simulink model "screening_stage1_pipeline"  (R2026a)
settings: Solver=VariableStepAuto
values from neighbouring files (symbols this model uses):
  m = result.lesionMasks.(code)    [runScreeningPipeline.m]
undefined symbols (not defined in the file or in its folder): n
settings Model: Creator=keert  LastModifiedBy=keert

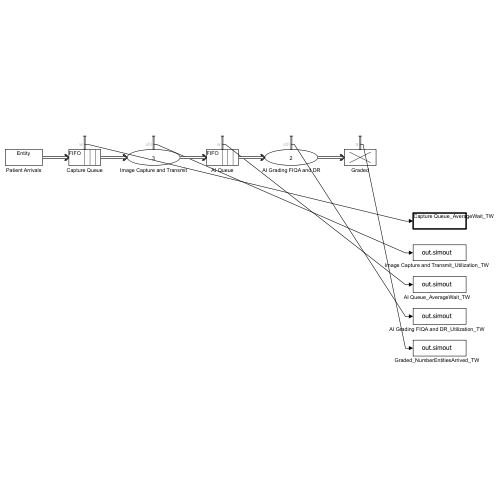
[thumbnail: Simulink's stored preview of the top-level diagram]
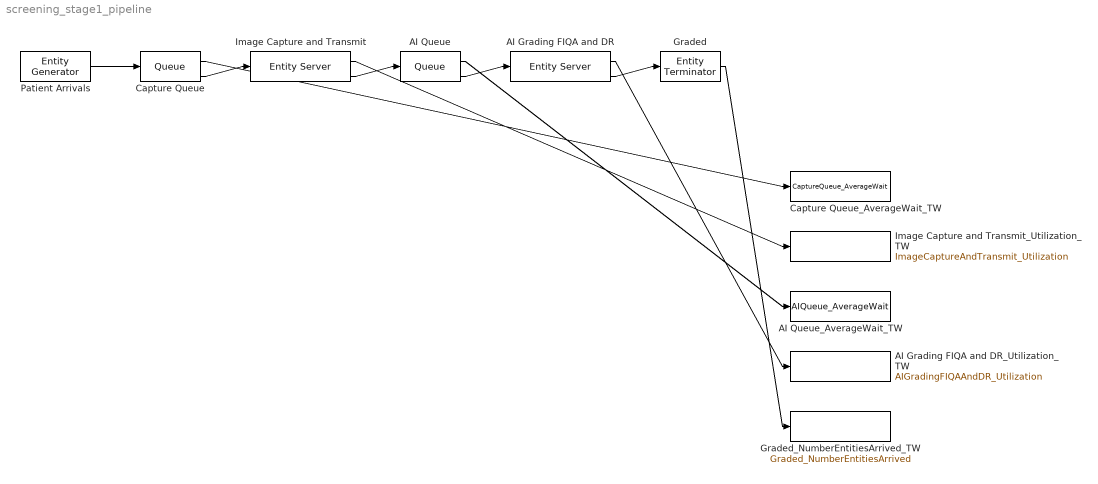
== system screening_stage1_pipeline ==
  AI Grading FIQA and DR : EntityServer  InputPortMessageModes=m  OutputPortMessageModes=n,m  Capacity=2  ServiceTimeValue=0.2  Utilization=on
      settings: OutputPortMap=o5,o9
  AI Grading FIQA and DR_Utilization_TW : ToWorkspace  VariableName=AIGradingFIQAAndDR_Utilization  SaveFormat=Structure  SampleTime=-1
  AI Queue : Queue  InputPortMessageModes=m  OutputPortMessageModes=n,m  AverageWait=on
      settings: OutputPortMap=o2,o5
  AI Queue_AverageWait_TW : ToWorkspace  VariableName=AIQueue_AverageWait  SaveFormat=Structure  SampleTime=-1
  Capture Queue : Queue  InputPortMessageModes=m  OutputPortMessageModes=n,m  AverageWait=on
      settings: OutputPortMap=o2,o5
  Capture Queue_AverageWait_TW : ToWorkspace  VariableName=CaptureQueue_AverageWait  SaveFormat=Structure  SampleTime=-1
  Graded : EntityTerminator  InputPortMessageModes=m  NumberEntitiesArrived=on
      settings: OutputPortMap=o0
  Graded_NumberEntitiesArrived_TW : ToWorkspace  VariableName=Graded_NumberEntitiesArrived  SaveFormat=Structure  SampleTime=-1
  Image Capture and Transmit : EntityServer  InputPortMessageModes=m  OutputPortMessageModes=n,m  Capacity=3  ServiceTimeValue=0.392  Utilization=on
      settings: OutputPortMap=o5,o9
  Image Capture and Transmit_Utilization_TW : ToWorkspace  VariableName=ImageCaptureAndTransmit_Utilization  SaveFormat=Structure  SampleTime=-1
  Patient Arrivals : EntityGenerator  OutputPortMessageModes=m  Period=72  EntityType=Structured  EntityTypeName=Entity
  wires:
  Capture Queue/1 -> Capture Queue_AverageWait_TW/1
  Image Capture and Transmit/1 -> Image Capture and Transmit_Utilization_TW/1
  AI Queue/1 -> AI Queue_AverageWait_TW/1
  AI Grading FIQA and DR/1 -> AI Grading FIQA and DR_Utilization_TW/1
  Graded/1 -> Graded_NumberEntitiesArrived_TW/1
  Patient Arrivals/1 -> Capture Queue/1
  Capture Queue/2 -> Image Capture and Transmit/1
  Image Capture and Transmit/2 -> AI Queue/1
  AI Queue/2 -> AI Grading FIQA and DR/1
  AI Grading FIQA and DR/2 -> Graded/1
